simulink model "ctrl_TAPM"  (R2015a)
settings: Solver=ode3  StartTime=0.0  StopTime=inf  FixedStep=0.01  RelTol=1e-3
undefined symbols (not defined in the file): C, D, eps_c, epsilon, hd, hd2, I_s, k_cc, K_omega, K_q1f, K_q1r, K_q2f, K_q2r, K_q3f, K_q3r, K_q4f, K_q4r, K_q5f, K_q5r, K_q6f, K_q6r, K_T1f, K_T1r, K_T2f, K_T2r, K_T3f, K_T3r, K_T4f, K_T4r, K_T5f, K_T5r, K_T6f, K_T6r, Kp, Max_Acceleration, Max_rotation, Max_thrust, Min_thrust, n_c, n_max, p_cc, pwm_thr1_backward, pwm_thr1_forward, pwm_thr2_backward, pwm_thr2_forward, pwm_thr3_backward, pwm_thr3_forward, pwm_thr4_backward, pwm_thr4_forward, pwm_thr5_backward, pwm_thr5_forward, pwm_thr6_backward, pwm_thr6_forward, Q_f0, Q_max, r_cc, Rho, Thruster
libraries: marine_gnc x10, simulink x6, simulink_extras x3
(part 3 of 5)

== system ctrl_TAPM/Thruster control  ==
  "Desired thrust and angle " : Inport
  Delay : Delay  DelayLength=1  InitialCondition=0
  Demux : Demux  Outputs=12
  Mapping shaft speed and thrust : Selector  InputPortWidth=12  Indices="[1 7 2  8 3 9 4 10 5 11 6 12]"
  Mux : Mux  Inputs=12
  Mux1 : Mux  Inputs=2
  Selecting Desired thrust1 : Selector  InputPortWidth=12  Indices=[7 8 9 10 11 12]
  Selecting actual angle : Selector  InputPortWidth=12  Indices=[1 2 3 4 5 6]
  Subsystem1 : Subsystem
  Thrust and Shaft speed mapped to PWM : Subsystem
  Thruster 1 : Subsystem
      settings: AttributesFormatString=%<MinAlgLoopOccurrences>
  Thruster 2 : Subsystem
      settings: AttributesFormatString=%<MinAlgLoopOccurrences>
  Thruster 3 : Subsystem
      settings: AttributesFormatString=%<MinAlgLoopOccurrences>
  Thruster 4 : Subsystem
      settings: AttributesFormatString=%<MinAlgLoopOccurrences>
  Thruster 5 : Subsystem
      settings: AttributesFormatString=%<MinAlgLoopOccurrences>
  Thruster 6 : Subsystem
      settings: AttributesFormatString=%<MinAlgLoopOccurrences>
  "Commanded pwm " : Outport
  Commanded angle : Outport  Port=2
  Commanded thrust : Outport  Port=3
  wires:
  Selecting actual angle/1 -> Subsystem1/1(Calculated angles)
  "Desired thrust and angle "/1 -> Selecting actual angle/1, Selecting Desired thrust1/1
  Subsystem1/1(Commanded angles) -> Commanded angle/1
  Thrust and Shaft speed mapped to PWM/1(pwm) -> "Commanded pwm "/1
  Thrust and Shaft speed mapped to PWM/2(Force) -> Commanded thrust/1
  Thrust and Shaft speed mapped to PWM/3("Shaft speed ") -> Delay/1
  Thruster 1/1("Commanded thrust ") -> Mux/1
  Mux/1 -> Thrust and Shaft speed mapped to PWM/1(Calculated thrust)
  Mux1/1 -> Mapping shaft speed and thrust/1
  Delay/1 -> Mux1/2
  Mapping shaft speed and thrust/1 -> Demux/1
  Thruster 1/2(Shaft speed) -> Mux/2
  Demux/2 -> Thruster 1/2(shaft speed)
  Demux/1 -> Thruster 1/1(Desired thrust 1)
  Thruster 2/1("Commanded thrust ") -> Mux/3
  Demux/3 -> Thruster 2/1(Desired thrust 1)
  Demux/4 -> Thruster 2/2(shaft speed)
  Demux/5 -> Thruster 3/1(Desired thrust 1)
  Demux/6 -> Thruster 3/2(shaft speed)
  Demux/7 -> Thruster 4/1(Desired thrust 1)
  Demux/8 -> Thruster 4/2(shaft speed)
  Demux/9 -> Thruster 5/1(Desired thrust 1)
  Demux/10 -> Thruster 5/2(shaft speed)
  Demux/11 -> Thruster 6/1(Desired thrust 1)
  Demux/12 -> Thruster 6/2(shaft speed)
  Thruster 2/2(Shaft speed) -> Mux/4
  Thruster 3/1("Commanded thrust ") -> Mux/5
  Thruster 3/2(Shaft speed) -> Mux/6
  Thruster 4/1("Commanded thrust ") -> Mux/7
  Thruster 4/2(Shaft speed) -> Mux/8
  Thruster 5/1("Commanded thrust ") -> Mux/9
  Thruster 5/2(Shaft speed) -> Mux/10
  Thruster 6/1("Commanded thrust ") -> Mux/11
  Thruster 6/2(Shaft speed) -> Mux/12
  Selecting Desired thrust1/1 -> Mux1/1

== system ctrl_TAPM/Thruster measurment ==
  Mux1 : Mux  Inputs=6
  thr_angle_1 : S-Function  Priority=1  FunctionName=NIVeriStandIO  Parameters=width dtype portnum stime stype btype  mask(NI VeriStand Inport){portnum=1, width=-1, stime=-1, dtype=auto, stype=auto, btype=1}
      mask prompts: portnum "Port number:"; width "Port dimensions (-1 for dynamically sized):"; stime "Sample time (-1 for inherited):"; dtype "Data type:"; stype "Signal type:"; btype "Block type:"
      mask help: Use this inport on any level of nested subsystems to allow NI VeriStand software to map signals to it.
      mask init:
      | NIVeriStandIO_init;
      settings: CopyFcn=NIVeriStand_MDL_functions('', 'IO_copy');  DeleteFcn=NIVeriStand_MDL_functions('', 'IO_delete');  MoveFcn=set_param(gcb, 'Mask', 'on');
      mask Callback portnum: NIVeriStand_MDL_functions('', 'IO_setportnum');
      mask TypeOptions dtype: auto | double | single | int8 | uint8 | int16 | uint16 | int32 | uint32 | boolean
      mask Callback dtype: NIVeriStand_MDL_functions('', 'IO_booleansignal');
      mask TypeOptions stype: auto | real | complex
      mask Display:
      | patch([-x x], [-y y], [.90980 .81960 .32156]);
      | plot([xrad -x x xrad], [yrad -y y yrad]);
      | fprintf('NI In%d', portnum);
  thr_angle_2 : S-Function  Priority=2  FunctionName=NIVeriStandIO  Parameters=width dtype portnum stime stype btype  mask(NI VeriStand Inport){portnum=2, width=-1, stime=-1, dtype=auto, stype=auto, btype=1}
      mask prompts: portnum "Port number:"; width "Port dimensions (-1 for dynamically sized):"; stime "Sample time (-1 for inherited):"; dtype "Data type:"; stype "Signal type:"; btype "Block type:"
      mask help: Use this inport on any level of nested subsystems to allow NI VeriStand software to map signals to it.
      mask init:
      | NIVeriStandIO_init;
      settings: CopyFcn=NIVeriStand_MDL_functions('', 'IO_copy');  DeleteFcn=NIVeriStand_MDL_functions('', 'IO_delete');  MoveFcn=set_param(gcb, 'Mask', 'on');
      mask Callback portnum: NIVeriStand_MDL_functions('', 'IO_setportnum');
      mask TypeOptions dtype: auto | double | single | int8 | uint8 | int16 | uint16 | int32 | uint32 | boolean
      mask Callback dtype: NIVeriStand_MDL_functions('', 'IO_booleansignal');
      mask TypeOptions stype: auto | real | complex
      mask Display:
      | patch([-x x], [-y y], [.90980 .81960 .32156]);
      | plot([xrad -x x xrad], [yrad -y y yrad]);
      | fprintf('NI In%d', portnum);
  thr_angle_3 : S-Function  Priority=3  FunctionName=NIVeriStandIO  Parameters=width dtype portnum stime stype btype  mask(NI VeriStand Inport){portnum=3, width=-1, stime=-1, dtype=auto, stype=auto, btype=1}
      mask prompts: portnum "Port number:"; width "Port dimensions (-1 for dynamically sized):"; stime "Sample time (-1 for inherited):"; dtype "Data type:"; stype "Signal type:"; btype "Block type:"
      mask help: Use this inport on any level of nested subsystems to allow NI VeriStand software to map signals to it.
      mask init:
      | NIVeriStandIO_init;
      settings: CopyFcn=NIVeriStand_MDL_functions('', 'IO_copy');  DeleteFcn=NIVeriStand_MDL_functions('', 'IO_delete');  MoveFcn=set_param(gcb, 'Mask', 'on');
      mask Callback portnum: NIVeriStand_MDL_functions('', 'IO_setportnum');
      mask TypeOptions dtype: auto | double | single | int8 | uint8 | int16 | uint16 | int32 | uint32 | boolean
      mask Callback dtype: NIVeriStand_MDL_functions('', 'IO_booleansignal');
      mask TypeOptions stype: auto | real | complex
      mask Display:
      | patch([-x x], [-y y], [.90980 .81960 .32156]);
      | plot([xrad -x x xrad], [yrad -y y yrad]);
      | fprintf('NI In%d', portnum);
  thr_angle_4 : S-Function  Priority=4  FunctionName=NIVeriStandIO  Parameters=width dtype portnum stime stype btype  mask(NI VeriStand Inport){portnum=4, width=-1, stime=-1, dtype=auto, stype=auto, btype=1}
      mask prompts: portnum "Port number:"; width "Port dimensions (-1 for dynamically sized):"; stime "Sample time (-1 for inherited):"; dtype "Data type:"; stype "Signal type:"; btype "Block type:"
      mask help: Use this inport on any level of nested subsystems to allow NI VeriStand software to map signals to it.
      mask init:
      | NIVeriStandIO_init;
      settings: CopyFcn=NIVeriStand_MDL_functions('', 'IO_copy');  DeleteFcn=NIVeriStand_MDL_functions('', 'IO_delete');  MoveFcn=set_param(gcb, 'Mask', 'on');
      mask Callback portnum: NIVeriStand_MDL_functions('', 'IO_setportnum');
      mask TypeOptions dtype: auto | double | single | int8 | uint8 | int16 | uint16 | int32 | uint32 | boolean
      mask Callback dtype: NIVeriStand_MDL_functions('', 'IO_booleansignal');
      mask TypeOptions stype: auto | real | complex
      mask Display:
      | patch([-x x], [-y y], [.90980 .81960 .32156]);
      | plot([xrad -x x xrad], [yrad -y y yrad]);
      | fprintf('NI In%d', portnum);
  thr_angle_5 : S-Function  Priority=5  FunctionName=NIVeriStandIO  Parameters=width dtype portnum stime stype btype  mask(NI VeriStand Inport){portnum=5, width=-1, stime=-1, dtype=auto, stype=auto, btype=1}
      mask prompts: portnum "Port number:"; width "Port dimensions (-1 for dynamically sized):"; stime "Sample time (-1 for inherited):"; dtype "Data type:"; stype "Signal type:"; btype "Block type:"
      mask help: Use this inport on any level of nested subsystems to allow NI VeriStand software to map signals to it.
      mask init:
      | NIVeriStandIO_init;
      settings: CopyFcn=NIVeriStand_MDL_functions('', 'IO_copy');  DeleteFcn=NIVeriStand_MDL_functions('', 'IO_delete');  MoveFcn=set_param(gcb, 'Mask', 'on');
      mask Callback portnum: NIVeriStand_MDL_functions('', 'IO_setportnum');
      mask TypeOptions dtype: auto | double | single | int8 | uint8 | int16 | uint16 | int32 | uint32 | boolean
      mask Callback dtype: NIVeriStand_MDL_functions('', 'IO_booleansignal');
      mask TypeOptions stype: auto | real | complex
      mask Display:
      | patch([-x x], [-y y], [.90980 .81960 .32156]);
      | plot([xrad -x x xrad], [yrad -y y yrad]);
      | fprintf('NI In%d', portnum);
  thr_angle_6 : S-Function  Priority=6  FunctionName=NIVeriStandIO  Parameters=width dtype portnum stime stype btype  mask(NI VeriStand Inport){portnum=6, width=-1, stime=-1, dtype=auto, stype=auto, btype=1}
      mask prompts: portnum "Port number:"; width "Port dimensions (-1 for dynamically sized):"; stime "Sample time (-1 for inherited):"; dtype "Data type:"; stype "Signal type:"; btype "Block type:"
      mask help: Use this inport on any level of nested subsystems to allow NI VeriStand software to map signals to it.
      mask init:
      | NIVeriStandIO_init;
      settings: CopyFcn=NIVeriStand_MDL_functions('', 'IO_copy');  DeleteFcn=NIVeriStand_MDL_functions('', 'IO_delete');  MoveFcn=set_param(gcb, 'Mask', 'on');
      mask Callback portnum: NIVeriStand_MDL_functions('', 'IO_setportnum');
      mask TypeOptions dtype: auto | double | single | int8 | uint8 | int16 | uint16 | int32 | uint32 | boolean
      mask Callback dtype: NIVeriStand_MDL_functions('', 'IO_booleansignal');
      mask TypeOptions stype: auto | real | complex
      mask Display:
      | patch([-x x], [-y y], [.90980 .81960 .32156]);
      | plot([xrad -x x xrad], [yrad -y y yrad]);
      | fprintf('NI In%d', portnum);
  alpha_m : Outport
  wires:
  thr_angle_3/1 -> Mux1/3
  thr_angle_1/1 -> Mux1/1
  Mux1/1 -> alpha_m/1
  thr_angle_5/1 -> Mux1/5
  thr_angle_4/1 -> Mux1/4
  thr_angle_6/1 -> Mux1/6
  thr_angle_2/1 -> Mux1/2

== system ctrl_TAPM/IMU/Wild point cleaner ==
  Y : Inport
  MATLAB Function : MATLAB Function  TreatAsAtomicUnit=on
  Memory : Memory  X0=[4.968, 4.965, 4.97, 4.975, 4.96]
  Memory1 : Memory  X0=[0, 0, 0, 0, 0, 0, 0]
  Y_filtered : Outport
  wires:
  Y/1 -> MATLAB Function/2(Y)
  MATLAB Function/2(Y_filtered) -> Memory1/1, Y_filtered/1
  MATLAB Function/1(V_hist1) -> Memory/1
  Memory/1 -> MATLAB Function/1(V_hist)
  Memory1/1 -> MATLAB Function/3(Y_prev)

== system ctrl_TAPM/IMU/Wild point cleaner1 ==
  Y : Inport
  MATLAB Function : MATLAB Function  TreatAsAtomicUnit=on
  Memory : Memory  X0=[4.968, 4.965, 4.97, 4.975, 4.96]
  Memory1 : Memory  X0=[0, 0, 0, 0, 0, 0, 0]
  Y_filtered : Outport
  wires:
  Y/1 -> MATLAB Function/2(Y)
  MATLAB Function/2(Y_filtered) -> Memory1/1, Y_filtered/1
  MATLAB Function/1(V_hist1) -> Memory/1
  Memory/1 -> MATLAB Function/1(V_hist)
  Memory1/1 -> MATLAB Function/3(Y_prev)

== system ctrl_TAPM/TAPM Controller w_observer/LQR ==
  SP : Inport
  eta : Inport  Port=2
  bias : Inport  Port=3
  Constant : Constant
  Delay : Delay  DelayLength=1  InitialCondition=0
  Integrator : Integrator  ExternalReset=rising  IgnoreLimit=on
  MATLAB Function : MATLAB Function  TreatAsAtomicUnit=on
  MATLAB Function1 : MATLAB Function  TreatAsAtomicUnit=on
  MATLAB Function2 : MATLAB Function  TreatAsAtomicUnit=on
  MATLAB Function3 : MATLAB Function  TreatAsAtomicUnit=on
  Multiport Switch : MultiPortSwitch  Inputs=2
  controller : S-Function  Priority=1  FunctionName=NIVeriStandIO  Parameters=width dtype portnum stime stype btype  mask(NI VeriStand Outport){portnum=1, width=-1, stime=-1, dtype=auto, stype=auto, btype=0}
      mask prompts: portnum "Port number:"; width "Port dimensions (-1 for dynamically sized):"; stime "Sample time (-1 for inherited):"; dtype "Data type:"; stype "Signal type:"; btype "Block type:"
      mask help: Use this outport on any level of nested subsystems to allow NI VeriStand software to map signals to it.
      mask init:
      | NIVeriStandIO_init;
      settings: CopyFcn=NIVeriStand_MDL_functions('', 'IO_copy');  DeleteFcn=NIVeriStand_MDL_functions('', 'IO_delete');  MoveFcn=set_param(gcb, 'Mask', 'on');
      mask Callback portnum: NIVeriStand_MDL_functions('', 'IO_setportnum');
      mask TypeOptions dtype: auto | double | single | int8 | uint8 | int16 | uint16 | int32 | uint32 | boolean
      mask Callback dtype: NIVeriStand_MDL_functions('', 'IO_booleansignal');
      mask TypeOptions stype: auto | real | complex
      mask Display:
      | patch([-x x], [-y y], [.90980 .81960 .32156]);
      | plot([xrad -x x xrad], [yrad -y y yrad]);
      | fprintf('NI Out%d', portnum);
  timer : S-Function  Priority=2  FunctionName=NIVeriStandIO  Parameters=width dtype portnum stime stype btype  mask(NI VeriStand Outport){portnum=2, width=-1, stime=-1, dtype=auto, stype=auto, btype=0}
      mask prompts: portnum "Port number:"; width "Port dimensions (-1 for dynamically sized):"; stime "Sample time (-1 for inherited):"; dtype "Data type:"; stype "Signal type:"; btype "Block type:"
      mask help: Use this outport on any level of nested subsystems to allow NI VeriStand software to map signals to it.
      mask init:
      | NIVeriStandIO_init;
      settings: CopyFcn=NIVeriStand_MDL_functions('', 'IO_copy');  DeleteFcn=NIVeriStand_MDL_functions('', 'IO_delete');  MoveFcn=set_param(gcb, 'Mask', 'on');
      mask Callback portnum: NIVeriStand_MDL_functions('', 'IO_setportnum');
      mask TypeOptions dtype: auto | double | single | int8 | uint8 | int16 | uint16 | int32 | uint32 | boolean
      mask Callback dtype: NIVeriStand_MDL_functions('', 'IO_booleansignal');
      mask TypeOptions stype: auto | real | complex
      mask Display:
      | patch([-x x], [-y y], [.90980 .81960 .32156]);
      | plot([xrad -x x xrad], [yrad -y y yrad]);
      | fprintf('NI Out%d', portnum);
  tau_d : Outport  PortDimensions=3
  wires:
  SP/1 -> MATLAB Function3/1(r), MATLAB Function1/1(r)
  eta/1 -> MATLAB Function/3(eta), MATLAB Function1/2(x_hat), MATLAB Function3/2(x_hat)
  Constant/1 -> Integrator/1
  MATLAB Function/1(reset) -> Integrator/2
  Integrator/1 -> Delay/1
  MATLAB Function/2(y) -> controller/1, Multiport Switch/1
  Delay/1 -> timer/1, MATLAB Function/1(timer)
  bias/1 -> MATLAB Function1/3(bias), MATLAB Function3/3(bias)
  [r_max] -> MATLAB Function/2(rmax)
  Multiport Switch/1 -> MATLAB Function2/1(u)
  MATLAB Function1/1(tau) -> Multiport Switch/2
  MATLAB Function3/1(tau) -> Multiport Switch/3
  MATLAB Function2/1(y) -> tau_d/1

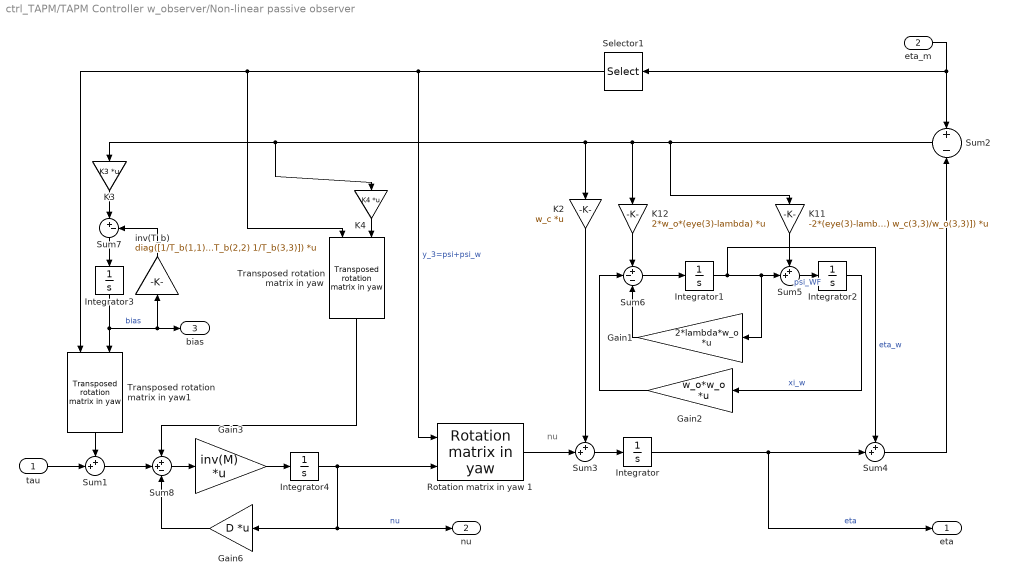
== system ctrl_TAPM/TAPM Controller w_observer/Non-linear passive observer  ==
  note: nu
  tau : Inport
  eta_m : Inport  Port=2
  Gain1 : Gain  Gain=2*lambda*w_o  Multiplication=Matrix(K*u)  SaturateOnIntegerOverflow=on  OutDataTypeStr=Inherit: Same as input  ParamDataTypeStr=Inherit: Same as input
  Gain2 : Gain  Gain=w_o*w_o  Multiplication=Matrix(K*u)  SaturateOnIntegerOverflow=on  OutDataTypeStr=Inherit: Same as input  ParamDataTypeStr=Inherit: Same as input
  Gain3 : Gain  Gain=inv(M)  Multiplication=Matrix(K*u)  SaturateOnIntegerOverflow=on  OutDataTypeStr=Inherit: Same as input  ParamDataTypeStr=Inherit: Same as input
  Gain6 : Gain  Gain=D  Multiplication=Matrix(K*u)  SaturateOnIntegerOverflow=on  OutDataTypeStr=Inherit: Same as input  ParamDataTypeStr=Inherit: Same as input
  Integrator : Integrator  InitialCondition=[0,0,0]'
  Integrator1 : Integrator
  Integrator2 : Integrator
  Integrator3 : Integrator
  Integrator4 : Integrator  InitialCondition=[0,0,0]'
  K11 : Gain  Gain=-2*(eye(3)-lambda)*diag([w_c(1,1)/w_o(1,1) w_c(2,2)/w_o(2,2) w_c(3,3)/w_o(3,3)])  Multiplication=Matrix(K*u)  SaturateOnIntegerOverflow=on  OutDataTypeStr=Inherit: Same as input  ParamDataTypeStr=Inherit: Same as input
  K12 : Gain  Gain=2*w_o*(eye(3)-lambda)  Multiplication=Matrix(K*u)  SaturateOnIntegerOverflow=on  OutDataTypeStr=Inherit: Same as input  ParamDataTypeStr=Inherit: Same as input
  K2 : Gain  Gain=w_c  Multiplication=Matrix(K*u)  SaturateOnIntegerOverflow=on  OutDataTypeStr=Inherit: Same as input  ParamDataTypeStr=Inherit: Same as input
  K3 : Gain  Gain=K3  Multiplication=Matrix(K*u)  SaturateOnIntegerOverflow=on  OutDataTypeStr=Inherit: Same as input  ParamDataTypeStr=Inherit: Same as input
  K4 : Gain  Gain=K4  Multiplication=Matrix(K*u)  SaturateOnIntegerOverflow=on  OutDataTypeStr=Inherit: Same as input  ParamDataTypeStr=Inherit: Same as input
  Rotation matrix in yaw 1 : marine_gnc/Models/ Kinematics/Rotation matrix in yaw 
  Selector1 : Selector  InputPortWidth=3  Indices=[3]
  Sum{1,3..5} (4 alike) : Sum  Inputs=++|  SaturateOnIntegerOverflow=on  InputSameDT=on  OutDataTypeStr=Inherit: Same as first input
  Sum2 : Sum  Inputs=+|-  SaturateOnIntegerOverflow=on  InputSameDT=on  OutDataTypeStr=Inherit: Same as first input
  Sum6 : Sum  Inputs=+--  SaturateOnIntegerOverflow=on  InputSameDT=on  OutDataTypeStr=Inherit: Same as first input
  Sum7 : Sum  Inputs=|+-  SaturateOnIntegerOverflow=on  InputSameDT=on  OutDataTypeStr=Inherit: Same as first input
  Sum8 : Sum  Inputs=++-  SaturateOnIntegerOverflow=on  InputSameDT=on  OutDataTypeStr=Inherit: Same as first input
  Transposed rotation matrix in yaw : marine_gnc/Models/ Kinematics/Transposed rotation  matrix in yaw
  Transposed rotation matrix in yaw1 : marine_gnc/Models/ Kinematics/Transposed rotation  matrix in yaw
  inv(T_b) : Gain  Gain=diag([1/T_b(1,1) 1/T_b(2,2) 1/T_b(3,3)])  Multiplication=Matrix(K*u)  SaturateOnIntegerOverflow=on  OutDataTypeStr=Inherit: Same as input  ParamDataTypeStr=Inherit: Same as input
  eta : Outport
  nu : Outport  Port=2
  bias : Outport  Port=3  PortDimensions=3
  wires:
  Sum3/1 -> Integrator/1
  Integrator2/1 -> Gain2/1  "xi_w"
  Gain2/1 -> Sum6/2
  Sum6/1 -> Integrator1/1
  Sum4/1 -> Sum2/2
  Sum2/1 -> K4/1, K3/1, K2/1, K12/1, K11/1
  Gain1/1 -> Sum6/3
  K2/1 -> Sum3/1
  Integrator/1 -> Sum4/2, eta/1  "eta"
  inv(T_b)/1 -> Sum7/2
  Integrator3/1 -> Transposed rotation matrix in yaw1/2, bias/1, inv(T_b)/1  "bias"
  tau/1 -> Sum1/2
  Integrator1/1 -> Sum4/1, Gain1/1, Sum5/2  "eta_w"
  K12/1 -> Sum6/1
  K11/1 -> Sum5/1
  eta_m/1 -> Selector1/1, Sum2/1
  Sum5/1 -> Integrator2/1  "psi_WF"
  Sum7/1 -> Integrator3/1
  Sum1/1 -> Sum8/2
  Rotation matrix in yaw 1/1 -> Sum3/2
  K3/1 -> Sum7/1
  Selector1/1 -> Transposed rotation matrix in yaw1/1, Transposed rotation matrix in yaw/1, Rotation matrix in yaw 1/1  "y_3=psi+psi_w"
  Gain3/1 -> Integrator4/1
  Sum8/1 -> Gain3/1
  Integrator4/1 -> nu/1, Gain6/1, Rotation matrix in yaw 1/2  "nu"
  Transposed rotation matrix in yaw1/1 -> Sum1/1
  Transposed rotation matrix in yaw/1 -> Sum8/1
  K4/1 -> Transposed rotation matrix in yaw/2
  Gain6/1 -> Sum8/3

== system ctrl_TAPM/TAPM Controller w_observer/PID ==
  eta_ref : Inport
  eta : Inport  Port=2
  nu : Inport  Port=3
  Constant : Constant
  DP controller : Subsystem  AncestorBlock="marine_gnc/Control/Dynamic  Positioning /DP controller"
  DP controller1 : Subsystem  AncestorBlock="marine_gnc/Control/Dynamic  Positioning /DP controller"
  Delay : Delay  DelayLength=1  InitialCondition=0
  Integrator : Integrator  ExternalReset=rising  IgnoreLimit=on
  MATLAB Function : MATLAB Function  TreatAsAtomicUnit=on
  Multiport Switch : MultiPortSwitch  Inputs=2
  controller : S-Function  Priority=1  FunctionName=NIVeriStandIO  Parameters=width dtype portnum stime stype btype  mask(NI VeriStand Outport){portnum=1, width=-1, stime=-1, dtype=auto, stype=auto, btype=0}
      mask prompts: portnum "Port number:"; width "Port dimensions (-1 for dynamically sized):"; stime "Sample time (-1 for inherited):"; dtype "Data type:"; stype "Signal type:"; btype "Block type:"
      mask help: Use this outport on any level of nested subsystems to allow NI VeriStand software to map signals to it.
      mask init:
      | NIVeriStandIO_init;
      settings: CopyFcn=NIVeriStand_MDL_functions('', 'IO_copy');  DeleteFcn=NIVeriStand_MDL_functions('', 'IO_delete');  MoveFcn=set_param(gcb, 'Mask', 'on');
      mask Callback portnum: NIVeriStand_MDL_functions('', 'IO_setportnum');
      mask TypeOptions dtype: auto | double | single | int8 | uint8 | int16 | uint16 | int32 | uint32 | boolean
      mask Callback dtype: NIVeriStand_MDL_functions('', 'IO_booleansignal');
      mask TypeOptions stype: auto | real | complex
      mask Display:
      | patch([-x x], [-y y], [.90980 .81960 .32156]);
      | plot([xrad -x x xrad], [yrad -y y yrad]);
      | fprintf('NI Out%d', portnum);
  timer : S-Function  Priority=2  FunctionName=NIVeriStandIO  Parameters=width dtype portnum stime stype btype  mask(NI VeriStand Outport){portnum=2, width=-1, stime=-1, dtype=auto, stype=auto, btype=0}
      mask prompts: portnum "Port number:"; width "Port dimensions (-1 for dynamically sized):"; stime "Sample time (-1 for inherited):"; dtype "Data type:"; stype "Signal type:"; btype "Block type:"
      mask help: Use this outport on any level of nested subsystems to allow NI VeriStand software to map signals to it.
      mask init:
      | NIVeriStandIO_init;
      settings: CopyFcn=NIVeriStand_MDL_functions('', 'IO_copy');  DeleteFcn=NIVeriStand_MDL_functions('', 'IO_delete');  MoveFcn=set_param(gcb, 'Mask', 'on');
      mask Callback portnum: NIVeriStand_MDL_functions('', 'IO_setportnum');
      mask TypeOptions dtype: auto | double | single | int8 | uint8 | int16 | uint16 | int32 | uint32 | boolean
      mask Callback dtype: NIVeriStand_MDL_functions('', 'IO_booleansignal');
      mask TypeOptions stype: auto | real | complex
      mask Display:
      | patch([-x x], [-y y], [.90980 .81960 .32156]);
      | plot([xrad -x x xrad], [yrad -y y yrad]);
      | fprintf('NI Out%d', portnum);
  tau : Outport
  wires:
  DP controller/1(tau) -> Multiport Switch/2
  nu/1 -> DP controller1/3(nu), DP controller/3(nu)
  eta_ref/1 -> DP controller1/1(eta_ref), DP controller/1(eta_ref)
  eta/1 -> DP controller1/2(eta), MATLAB Function/3(eta), DP controller/2(eta)
  Constant/1 -> Integrator/1
  MATLAB Function/1(reset) -> Integrator/2
  Integrator/1 -> Delay/1
  MATLAB Function/2(y) -> controller/1, Multiport Switch/1
  Delay/1 -> timer/1, MATLAB Function/1(timer)
  [r_max] -> MATLAB Function/2(rmax)
  Multiport Switch/1 -> tau/1
  DP controller1/1(tau) -> Multiport Switch/3

== system ctrl_TAPM/TAPM Controller w_observer/SP Generator ==
  eta : Inport
  wave_dir : Inport  Port=2
  Constant1 : Constant  Value=pi
  Gain : Gain  Gain=diag([1/(1/sqrt(90)) 1/(1/sqrt(90))])  Multiplication=Matrix(K*u)
  Gain1 : Gain  Gain=diag([1/(1/sqrt(90)) 1/(1/sqrt(90))])  Multiplication=Matrix(K*u)
  Integrator : Integrator  InitialCondition=[0 0]
  Mux : Mux  Inputs=2
  Selector : Selector  InputPortWidth=3  Indices=[1 2]
  Set-Point Limiter : MATLAB Function  TreatAsAtomicUnit=on
  Sum : Sum  Inputs=|++
  Sum1 : Sum  Inputs=|+-
  Transfer Fcn2 : TransferFcn  Denominator=[0.5 1]
  SP : Outport  PortDimensions=3
  wires:
  Integrator/1 -> Gain/1, Set-Point Limiter/1(sp)
  [fzp] -> Set-Point Limiter/2(fzp)
  [r_max] -> Set-Point Limiter/3(rmax)
  Mux/1 -> SP/1
  eta/1 -> Selector/1
  Transfer Fcn2/1 -> Mux/2
  Constant1/1 -> Sum/1
  Sum/1 -> Transfer Fcn2/1
  wave_dir/1 -> Sum/2
  Set-Point Limiter/1(sp_new) -> Mux/1
  Sum1/1 -> Integrator/1
  Selector/1 -> Gain1/1
  Gain/1 -> Sum1/2
  Gain1/1 -> Sum1/1

== system ctrl_TAPM/Thrust allocation/Optimal angle path and constraints on rotation speed ==
  Desired Angle : Inport  Partition=on  PartitionDimension=1  PartitionWidth=1
  "initial angle " : Inport  Port=2  Partition=on  PartitionDimension=1  PartitionWidth=1
  reset : Inport  Port=3  Partition=on  PartitionDimension=1  PartitionWidth=1
  Degrees to Radians : simulink_extras/Transformations/Degrees to Radians
  Delay : Delay  DelayLength=1  InitialCondition=0
  Discrete-Time Integrator : DiscreteIntegrator  ExternalReset=either  InitialConditionSource=external  InitialConditionSetting=State (most efficient)  SampleTime=0.01
  Ensuring angle is [-pi pi] : MATLAB Function  TreatAsAtomicUnit=on
  For Each : ForEach  DisableCoverage=on  IndexMode=One-based
  MATLAB Function1 : MATLAB Function  TreatAsAtomicUnit=on
  Max Rotation Rate : Saturate  UpperLimit=Max_rotation  LowerLimit=-Max_rotation
  commanded Angle : Outport  ConcatenationDimension=1
  wires:
  Degrees to Radians/1 -> Ensuring angle is [-pi pi]/1(angle)
  Ensuring angle is [-pi pi]/1(y) -> commanded Angle/1
  Discrete-Time Integrator/1 -> Degrees to Radians/1, Delay/1  "angle"
  "initial angle "/1 -> Discrete-Time Integrator/3
  Max Rotation Rate/1 -> Discrete-Time Integrator/1
  MATLAB Function1/1(psi_D) -> Max Rotation Rate/1
  Desired Angle/1 -> MATLAB Function1/1(desired)
  reset/1 -> Discrete-Time Integrator/2
  Delay/1 -> MATLAB Function1/2(actual)

== system ctrl_TAPM/Thruster control /Subsystem1 ==
  Calculated angles : Inport
  Demux : Demux  Outputs=6
  Mux : Mux  Inputs=6
  Saturation {1..6} (6 alike) : Saturate  UpperLimit=pi  LowerLimit=-pi
  Commanded angles : Outport
  wires:
  Calculated angles/1 -> Demux/1
  Demux/1 -> Saturation 1/1
  Demux/2 -> Saturation 2/1
  Demux/3 -> Saturation 3/1
  Demux/4 -> Saturation 4/1
  Demux/5 -> Saturation 5/1
  Demux/6 -> Saturation 6/1
  Mux/1 -> Commanded angles/1
  Saturation 1/1 -> Mux/1
  Saturation 6/1 -> Mux/6
  Saturation 5/1 -> Mux/5
  Saturation 2/1 -> Mux/2
  Saturation 3/1 -> Mux/3
  Saturation 4/1 -> Mux/4

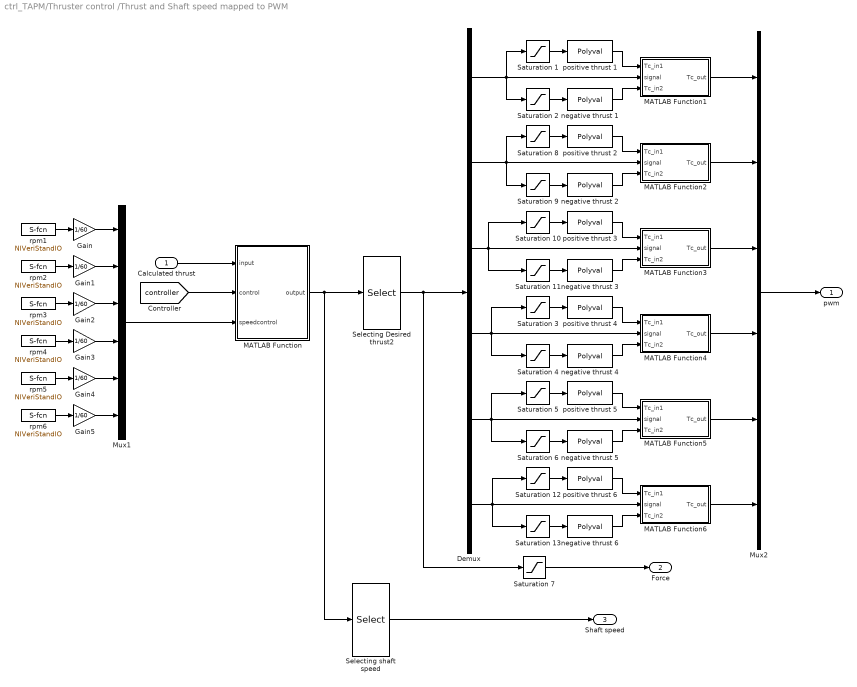
== system ctrl_TAPM/Thruster control /Thrust and Shaft speed mapped to PWM ==
  Calculated thrust : Inport
  Demux : Demux  Outputs=6
  Gain{,1..5} (6 alike) : Gain  Gain=1/60
  MATLAB Function : MATLAB Function  TreatAsAtomicUnit=on
  MATLAB Function1 : MATLAB Function  TreatAsAtomicUnit=on
  MATLAB Function2 : MATLAB Function  TreatAsAtomicUnit=on
  MATLAB Function3 : MATLAB Function  TreatAsAtomicUnit=on
  MATLAB Function4 : MATLAB Function  TreatAsAtomicUnit=on
  MATLAB Function5 : MATLAB Function  TreatAsAtomicUnit=on
  MATLAB Function6 : MATLAB Function  TreatAsAtomicUnit=on
  Mux1 : Mux  Inputs=6
  Mux2 : Mux  Inputs=6
  Saturation {1,3,5,8,10,12} (6 alike) : Saturate  UpperLimit=Max_thrust  LowerLimit=0
  Saturation {2,4,6,9,11,13} (6 alike) : Saturate  UpperLimit=0  LowerLimit=Min_thrust
  Saturation 7 : Saturate  UpperLimit=Max_thrust  LowerLimit=-Max_thrust
  Selecting Desired thrust2 : Selector  InputPortWidth=12  Indices=[1 3 5 7 9 11]
  Selecting shaft speed : Selector  InputPortWidth=12  Indices=[2 4 6 8 10 12]
  negative thrust 1 : Polyval  Coefs=pwm_thr1_backward
  negative thrust 2 : Polyval  Coefs=pwm_thr2_backward
  negative thrust 3 : Polyval  Coefs=pwm_thr3_backward
  negative thrust 4 : Polyval  Coefs=pwm_thr4_backward
  negative thrust 5 : Polyval  Coefs=pwm_thr5_backward
  negative thrust 6 : Polyval  Coefs=pwm_thr6_backward
  positive thrust 1 : Polyval  Coefs=pwm_thr1_forward
  positive thrust 2 : Polyval  Coefs=pwm_thr2_forward
  positive thrust 3 : Polyval  Coefs=pwm_thr3_forward
  positive thrust 4 : Polyval  Coefs=pwm_thr4_forward
  positive thrust 5 : Polyval  Coefs=pwm_thr5_forward
  positive thrust 6 : Polyval  Coefs=pwm_thr6_forward
  "rpm1 " : S-Function  Priority=1  FunctionName=NIVeriStandIO  Parameters=width dtype portnum stime stype btype  mask(NI VeriStand Inport){portnum=1, width=-1, stime=-1, dtype=auto, stype=auto, btype=1}
      mask prompts: portnum "Port number:"; width "Port dimensions (-1 for dynamically sized):"; stime "Sample time (-1 for inherited):"; dtype "Data type:"; stype "Signal type:"; btype "Block type:"
      mask help: Use this inport on any level of nested subsystems to allow NI VeriStand software to map signals to it.
      mask init:
      | NIVeriStandIO_init;
      settings: CopyFcn=NIVeriStand_MDL_functions('', 'IO_copy');  DeleteFcn=NIVeriStand_MDL_functions('', 'IO_delete');  MoveFcn=set_param(gcb, 'Mask', 'on');
      mask Callback portnum: NIVeriStand_MDL_functions('', 'IO_setportnum');
      mask TypeOptions dtype: auto | double | single | int8 | uint8 | int16 | uint16 | int32 | uint32 | boolean
      mask Callback dtype: NIVeriStand_MDL_functions('', 'IO_booleansignal');
      mask TypeOptions stype: auto | real | complex
      mask Display:
      | patch([-x x], [-y y], [.90980 .81960 .32156]);
      | plot([xrad -x x xrad], [yrad -y y yrad]);
      | fprintf('NI In%d', portnum);
  rpm2 : S-Function  Priority=2  FunctionName=NIVeriStandIO  Parameters=width dtype portnum stime stype btype  mask(NI VeriStand Inport){portnum=2, width=-1, stime=-1, dtype=auto, stype=auto, btype=1}
      mask prompts: portnum "Port number:"; width "Port dimensions (-1 for dynamically sized):"; stime "Sample time (-1 for inherited):"; dtype "Data type:"; stype "Signal type:"; btype "Block type:"
      mask help: Use this inport on any level of nested subsystems to allow NI VeriStand software to map signals to it.
      mask init:
      | NIVeriStandIO_init;
      settings: CopyFcn=NIVeriStand_MDL_functions('', 'IO_copy');  DeleteFcn=NIVeriStand_MDL_functions('', 'IO_delete');  MoveFcn=set_param(gcb, 'Mask', 'on');
      mask Callback portnum: NIVeriStand_MDL_functions('', 'IO_setportnum');
      mask TypeOptions dtype: auto | double | single | int8 | uint8 | int16 | uint16 | int32 | uint32 | boolean
      mask Callback dtype: NIVeriStand_MDL_functions('', 'IO_booleansignal');
      mask TypeOptions stype: auto | real | complex
      mask Display:
      | patch([-x x], [-y y], [.90980 .81960 .32156]);
      | plot([xrad -x x xrad], [yrad -y y yrad]);
      | fprintf('NI In%d', portnum);
  rpm3 : S-Function  Priority=3  FunctionName=NIVeriStandIO  Parameters=width dtype portnum stime stype btype  mask(NI VeriStand Inport){portnum=3, width=-1, stime=-1, dtype=auto, stype=auto, btype=1}
      mask prompts: portnum "Port number:"; width "Port dimensions (-1 for dynamically sized):"; stime "Sample time (-1 for inherited):"; dtype "Data type:"; stype "Signal type:"; btype "Block type:"
      mask help: Use this inport on any level of nested subsystems to allow NI VeriStand software to map signals to it.
      mask init:
      | NIVeriStandIO_init;
      settings: CopyFcn=NIVeriStand_MDL_functions('', 'IO_copy');  DeleteFcn=NIVeriStand_MDL_functions('', 'IO_delete');  MoveFcn=set_param(gcb, 'Mask', 'on');
      mask Callback portnum: NIVeriStand_MDL_functions('', 'IO_setportnum');
      mask TypeOptions dtype: auto | double | single | int8 | uint8 | int16 | uint16 | int32 | uint32 | boolean
      mask Callback dtype: NIVeriStand_MDL_functions('', 'IO_booleansignal');
      mask TypeOptions stype: auto | real | complex
      mask Display:
      | patch([-x x], [-y y], [.90980 .81960 .32156]);
      | plot([xrad -x x xrad], [yrad -y y yrad]);
      | fprintf('NI In%d', portnum);
  rpm4 : S-Function  Priority=4  FunctionName=NIVeriStandIO  Parameters=width dtype portnum stime stype btype  mask(NI VeriStand Inport){portnum=4, width=-1, stime=-1, dtype=auto, stype=auto, btype=1}
      mask prompts: portnum "Port number:"; width "Port dimensions (-1 for dynamically sized):"; stime "Sample time (-1 for inherited):"; dtype "Data type:"; stype "Signal type:"; btype "Block type:"
      mask help: Use this inport on any level of nested subsystems to allow NI VeriStand software to map signals to it.
      mask init:
      | NIVeriStandIO_init;
      settings: CopyFcn=NIVeriStand_MDL_functions('', 'IO_copy');  DeleteFcn=NIVeriStand_MDL_functions('', 'IO_delete');  MoveFcn=set_param(gcb, 'Mask', 'on');
      mask Callback portnum: NIVeriStand_MDL_functions('', 'IO_setportnum');
      mask TypeOptions dtype: auto | double | single | int8 | uint8 | int16 | uint16 | int32 | uint32 | boolean
      mask Callback dtype: NIVeriStand_MDL_functions('', 'IO_booleansignal');
      mask TypeOptions stype: auto | real | complex
      mask Display:
      | patch([-x x], [-y y], [.90980 .81960 .32156]);
      | plot([xrad -x x xrad], [yrad -y y yrad]);
      | fprintf('NI In%d', portnum);
  rpm5 : S-Function  Priority=5  FunctionName=NIVeriStandIO  Parameters=width dtype portnum stime stype btype  mask(NI VeriStand Inport){portnum=5, width=-1, stime=-1, dtype=auto, stype=auto, btype=1}
      mask prompts: portnum "Port number:"; width "Port dimensions (-1 for dynamically sized):"; stime "Sample time (-1 for inherited):"; dtype "Data type:"; stype "Signal type:"; btype "Block type:"
      mask help: Use this inport on any level of nested subsystems to allow NI VeriStand software to map signals to it.
      mask init:
      | NIVeriStandIO_init;
      settings: CopyFcn=NIVeriStand_MDL_functions('', 'IO_copy');  DeleteFcn=NIVeriStand_MDL_functions('', 'IO_delete');  MoveFcn=set_param(gcb, 'Mask', 'on');
      mask Callback portnum: NIVeriStand_MDL_functions('', 'IO_setportnum');
      mask TypeOptions dtype: auto | double | single | int8 | uint8 | int16 | uint16 | int32 | uint32 | boolean
      mask Callback dtype: NIVeriStand_MDL_functions('', 'IO_booleansignal');
      mask TypeOptions stype: auto | real | complex
      mask Display:
      | patch([-x x], [-y y], [.90980 .81960 .32156]);
      | plot([xrad -x x xrad], [yrad -y y yrad]);
      | fprintf('NI In%d', portnum);
  rpm6 : S-Function  Priority=6  FunctionName=NIVeriStandIO  Parameters=width dtype portnum stime stype btype  mask(NI VeriStand Inport){portnum=6, width=-1, stime=-1, dtype=auto, stype=auto, btype=1}
      mask prompts: portnum "Port number:"; width "Port dimensions (-1 for dynamically sized):"; stime "Sample time (-1 for inherited):"; dtype "Data type:"; stype "Signal type:"; btype "Block type:"
      mask help: Use this inport on any level of nested subsystems to allow NI VeriStand software to map signals to it.
      mask init:
      | NIVeriStandIO_init;
      settings: CopyFcn=NIVeriStand_MDL_functions('', 'IO_copy');  DeleteFcn=NIVeriStand_MDL_functions('', 'IO_delete');  MoveFcn=set_param(gcb, 'Mask', 'on');
      mask Callback portnum: NIVeriStand_MDL_functions('', 'IO_setportnum');
      mask TypeOptions dtype: auto | double | single | int8 | uint8 | int16 | uint16 | int32 | uint32 | boolean
      mask Callback dtype: NIVeriStand_MDL_functions('', 'IO_booleansignal');
      mask TypeOptions stype: auto | real | complex
      mask Display:
      | patch([-x x], [-y y], [.90980 .81960 .32156]);
      | plot([xrad -x x xrad], [yrad -y y yrad]);
      | fprintf('NI In%d', portnum);
  pwm : Outport
  Force : Outport  Port=2
  "Shaft speed " : Outport  Port=3
  wires:
  MATLAB Function/1(output) -> Selecting shaft speed/1, Selecting Desired thrust2/1
  [controller] -> MATLAB Function/2(control)
  Mux2/1 -> pwm/1
  Selecting Desired thrust2/1 -> Saturation 7/1, Demux/1
  Selecting shaft speed/1 -> "Shaft speed "/1
  Saturation 7/1 -> Force/1
  "rpm1 "/1 -> Gain/1
  rpm2/1 -> Gain1/1
  rpm3/1 -> Gain2/1
  rpm4/1 -> Gain3/1
  rpm5/1 -> Gain4/1
  rpm6/1 -> Gain5/1
  Mux1/1 -> MATLAB Function/3(speedcontrol)
  positive thrust 1/1 -> MATLAB Function1/1(Tc_in1)
  negative thrust 1/1 -> MATLAB Function1/3(Tc_in2)
  Demux/1 -> Saturation 1/1, MATLAB Function1/2(signal), Saturation 2/1
  MATLAB Function1/1(Tc_out) -> Mux2/1
  Saturation 1/1 -> positive thrust 1/1
  Saturation 2/1 -> negative thrust 1/1
  positive thrust 2/1 -> MATLAB Function2/1(Tc_in1)
  negative thrust 2/1 -> MATLAB Function2/3(Tc_in2)
  Demux/2 -> Saturation 9/1, Saturation 8/1, MATLAB Function2/2(signal)
  MATLAB Function2/1(Tc_out) -> Mux2/2
  Saturation 8/1 -> positive thrust 2/1
  Saturation 9/1 -> negative thrust 2/1
  positive thrust 3/1 -> MATLAB Function3/1(Tc_in1)
  negative thrust 3/1 -> MATLAB Function3/3(Tc_in2)
  Demux/3 -> Saturation 11/1, MATLAB Function3/2(signal), Saturation 10/1
  MATLAB Function3/1(Tc_out) -> Mux2/3
  Saturation 10/1 -> positive thrust 3/1
  Saturation 11/1 -> negative thrust 3/1
  positive thrust 4/1 -> MATLAB Function4/1(Tc_in1)
  negative thrust 4/1 -> MATLAB Function4/3(Tc_in2)
  MATLAB Function4/1(Tc_out) -> Mux2/4
  Saturation 3/1 -> positive thrust 4/1
  Saturation 4/1 -> negative thrust 4/1
  Demux/4 -> Saturation 3/1, Saturation 4/1, MATLAB Function4/2(signal)
  positive thrust 5/1 -> MATLAB Function5/1(Tc_in1)
  negative thrust 5/1 -> MATLAB Function5/3(Tc_in2)
  MATLAB Function5/1(Tc_out) -> Mux2/5
  Saturation 5/1 -> positive thrust 5/1
  Saturation 6/1 -> negative thrust 5/1
  Demux/5 -> Saturation 5/1, MATLAB Function5/2(signal), Saturation 6/1
  positive thrust 6/1 -> MATLAB Function6/1(Tc_in1)
  negative thrust 6/1 -> MATLAB Function6/3(Tc_in2)
  MATLAB Function6/1(Tc_out) -> Mux2/6
  Saturation 12/1 -> positive thrust 6/1
  Saturation 13/1 -> negative thrust 6/1
  Demux/6 -> Saturation 13/1, Saturation 12/1, MATLAB Function6/2(signal)
  Gain/1 -> Mux1/1
  Gain5/1 -> Mux1/6
  Gain4/1 -> Mux1/5
  Gain3/1 -> Mux1/4
  Gain2/1 -> Mux1/3
  Gain1/1 -> Mux1/2
  Calculated thrust/1 -> MATLAB Function/1(input)

== system ctrl_TAPM/Thruster control /Thruster 1 ==
  Desired thrust 1 : Inport
  shaft speed : Inport  Port=2
  Constant : Constant  Value=hd2.den{1,1}
  Constant1 : Constant  Value=hd2.num{1,1}
  Delay : Delay  DelayLength=1  InitialCondition=0
  Discrete Transfer Fcn : DiscreteTransferFcn  NumeratorSource=Input port  DenominatorSource=Input port  Denominator=[0.2 1]  SampleTime=0.01  a0EqualsOne=on
      settings: InputPortMap=u0,p1,p3
  Losses (placeholder) : Constant  Value=0
  Propeller Hydrodynamics : Subsystem
  Shaft dynamics : Subsystem
  Thruster control : Subsystem
  "Commanded thrust " : Outport
  Shaft speed : Outport  Port=2
  wires:
  Losses (placeholder)/1 -> Propeller Hydrodynamics/1(env)
  Shaft dynamics/1(n) -> Shaft speed/1, Propeller Hydrodynamics/2(n)
  Propeller Hydrodynamics/2(Qa) -> Delay/1
  Propeller Hydrodynamics/1(Ta) -> "Commanded thrust "/1
  Thruster control/1(Qc) -> Discrete Transfer Fcn/1
  Constant1/1 -> Discrete Transfer Fcn/2
  Constant/1 -> Discrete Transfer Fcn/3
  Discrete Transfer Fcn/1 -> Shaft dynamics/1(Qm)
  shaft speed/1 -> Thruster control/2(n)
  Delay/1 -> Shaft dynamics/2(Qa)
  Desired thrust 1/1 -> Thruster control/1("T_d ")

== system ctrl_TAPM/Thruster control /Thruster 2 ==
  Desired thrust 1 : Inport
  shaft speed : Inport  Port=2
  Constant : Constant  Value=hd2.den{1,1}
  Constant1 : Constant  Value=hd2.num{1,1}
  Delay : Delay  DelayLength=1  InitialCondition=0
  Discrete Transfer Fcn : DiscreteTransferFcn  NumeratorSource=Input port  DenominatorSource=Input port  Denominator=[0.2 1]  SampleTime=0.01  a0EqualsOne=on
      settings: InputPortMap=u0,p1,p3
  Losses (placeholder) : Constant  Value=0
  Propeller Hydrodynamics : Subsystem
  Shaft dynamics : Subsystem
  Thruster control : Subsystem
  "Commanded thrust " : Outport
  Shaft speed : Outport  Port=2
  wires:
  Losses (placeholder)/1 -> Propeller Hydrodynamics/1(env)
  Shaft dynamics/1(n) -> Propeller Hydrodynamics/2(n), Shaft speed/1
  Propeller Hydrodynamics/2(Qa) -> Delay/1
  Thruster control/1(Qc) -> Discrete Transfer Fcn/1
  Discrete Transfer Fcn/1 -> Shaft dynamics/1(Qm)
  Desired thrust 1/1 -> Thruster control/1("T_d ")
  Propeller Hydrodynamics/1(Ta) -> "Commanded thrust "/1
  Constant1/1 -> Discrete Transfer Fcn/2
  Constant/1 -> Discrete Transfer Fcn/3
  shaft speed/1 -> Thruster control/2(n)
  Delay/1 -> Shaft dynamics/2(Qa)

== system ctrl_TAPM/Thruster control /Thruster 3 ==
  Desired thrust 1 : Inport
  shaft speed : Inport  Port=2
  Constant : Constant  Value=hd2.den{1,1}
  Constant1 : Constant  Value=hd2.num{1,1}
  Delay : Delay  DelayLength=1  InitialCondition=0
  Discrete Transfer Fcn : DiscreteTransferFcn  NumeratorSource=Input port  DenominatorSource=Input port  Denominator=[0.2 1]  SampleTime=0.01  a0EqualsOne=on
      settings: InputPortMap=u0,p1,p3
  Losses (placeholder) : Constant  Value=0
  Propeller Hydrodynamics : Subsystem
  Shaft dynamics : Subsystem
  Thruster control : Subsystem
  "Commanded thrust " : Outport
  Shaft speed : Outport  Port=2
  wires:
  Losses (placeholder)/1 -> Propeller Hydrodynamics/1(env)
  Shaft dynamics/1(n) -> Propeller Hydrodynamics/2(n), Shaft speed/1
  Propeller Hydrodynamics/2(Qa) -> Delay/1
  Thruster control/1(Qc) -> Discrete Transfer Fcn/1
  Discrete Transfer Fcn/1 -> Shaft dynamics/1(Qm)
  Desired thrust 1/1 -> Thruster control/1("T_d ")
  Propeller Hydrodynamics/1(Ta) -> "Commanded thrust "/1
  Constant1/1 -> Discrete Transfer Fcn/2
  Constant/1 -> Discrete Transfer Fcn/3
  shaft speed/1 -> Thruster control/2(n)
  Delay/1 -> Shaft dynamics/2(Qa)

== system ctrl_TAPM/Thruster control /Thruster 4 ==
  Desired thrust 1 : Inport
  shaft speed : Inport  Port=2
  Constant : Constant  Value=hd2.den{1,1}
  Constant1 : Constant  Value=hd2.num{1,1}
  Delay : Delay  DelayLength=1  InitialCondition=0
  Discrete Transfer Fcn : DiscreteTransferFcn  NumeratorSource=Input port  DenominatorSource=Input port  Denominator=[0.2 1]  SampleTime=0.01  a0EqualsOne=on
      settings: InputPortMap=u0,p1,p3
  Losses (placeholder) : Constant  Value=0
  Propeller Hydrodynamics : Subsystem
  Shaft dynamics : Subsystem
  Thruster control : Subsystem
  "Commanded thrust " : Outport
  Shaft speed : Outport  Port=2
  wires:
  Losses (placeholder)/1 -> Propeller Hydrodynamics/1(env)
  Shaft dynamics/1(n) -> Propeller Hydrodynamics/2(n), Shaft speed/1
  Propeller Hydrodynamics/2(Qa) -> Delay/1
  Thruster control/1(Qc) -> Discrete Transfer Fcn/1
  Discrete Transfer Fcn/1 -> Shaft dynamics/1(Qm)
  Desired thrust 1/1 -> Thruster control/1("T_d ")
  Propeller Hydrodynamics/1(Ta) -> "Commanded thrust "/1
  Constant1/1 -> Discrete Transfer Fcn/2
  Constant/1 -> Discrete Transfer Fcn/3
  shaft speed/1 -> Thruster control/2(n)
  Delay/1 -> Shaft dynamics/2(Qa)

== system ctrl_TAPM/Thruster control /Thruster 5 ==
  Desired thrust 1 : Inport
  shaft speed : Inport  Port=2
  Constant : Constant  Value=hd2.den{1,1}
  Constant1 : Constant  Value=hd2.num{1,1}
  Delay : Delay  DelayLength=1  InitialCondition=0
  Discrete Transfer Fcn : DiscreteTransferFcn  NumeratorSource=Input port  DenominatorSource=Input port  Denominator=[0.2 1]  SampleTime=0.01  a0EqualsOne=on
      settings: InputPortMap=u0,p1,p3
  Losses (placeholder) : Constant  Value=0
  Propeller Hydrodynamics : Subsystem
  Shaft dynamics : Subsystem
  Thruster control : Subsystem
  "Commanded thrust " : Outport
  Shaft speed : Outport  Port=2
  wires:
  Losses (placeholder)/1 -> Propeller Hydrodynamics/1(env)
  Shaft dynamics/1(n) -> Propeller Hydrodynamics/2(n), Shaft speed/1
  Propeller Hydrodynamics/2(Qa) -> Delay/1
  Thruster control/1(Qc) -> Discrete Transfer Fcn/1
  Discrete Transfer Fcn/1 -> Shaft dynamics/1(Qm)
  Desired thrust 1/1 -> Thruster control/1("T_d ")
  Propeller Hydrodynamics/1(Ta) -> "Commanded thrust "/1
  Constant1/1 -> Discrete Transfer Fcn/2
  Constant/1 -> Discrete Transfer Fcn/3
  shaft speed/1 -> Thruster control/2(n)
  Delay/1 -> Shaft dynamics/2(Qa)

== system ctrl_TAPM/Thruster control /Thruster 6 ==
  Desired thrust 1 : Inport
  shaft speed : Inport  Port=2
  Constant : Constant  Value=hd2.den{1,1}
  Constant1 : Constant  Value=hd2.num{1,1}
  Delay : Delay  DelayLength=1  InitialCondition=0
  Discrete Transfer Fcn : DiscreteTransferFcn  NumeratorSource=Input port  DenominatorSource=Input port  Denominator=[0.2 1]  SampleTime=0.01  a0EqualsOne=on
      settings: InputPortMap=u0,p1,p3
  Losses (placeholder) : Constant  Value=0
  Propeller Hydrodynamics : Subsystem
  Shaft dynamics : Subsystem
  Thruster control : Subsystem
  "Commanded thrust " : Outport
  Shaft speed : Outport  Port=2
  wires:
  Losses (placeholder)/1 -> Propeller Hydrodynamics/1(env)
  Shaft dynamics/1(n) -> Propeller Hydrodynamics/2(n), Shaft speed/1
  Propeller Hydrodynamics/2(Qa) -> Delay/1
  Thruster control/1(Qc) -> Discrete Transfer Fcn/1
  Discrete Transfer Fcn/1 -> Shaft dynamics/1(Qm)
  Desired thrust 1/1 -> Thruster control/1("T_d ")
  Propeller Hydrodynamics/1(Ta) -> "Commanded thrust "/1
  Constant1/1 -> Discrete Transfer Fcn/2
  Constant/1 -> Discrete Transfer Fcn/3
  shaft speed/1 -> Thruster control/2(n)
  Delay/1 -> Shaft dynamics/2(Qa)

== system ctrl_TAPM/TAPM Controller w_observer/PID/DP controller ==
  eta_ref : Inport
  eta : Inport  Port=2
  nu : Inport  Port=3
  Demux : Demux  Outputs=3
  Integrator : Integrator
  Matrix Multiply : Product  Multiplication=Matrix(*)
  Matrix Multiply1 : Product  Multiplication=Matrix(*)
  Matrix Multiply2 : Product  Multiplication=Matrix(*)
  Mux : Mux  Inputs=3
  Sum1 : Sum  Inputs=|+-  SaturateOnIntegerOverflow=on  InputSameDT=on  OutDataTypeStr=Inherit: Same as first input
  Sum2 : Sum  Inputs=+-|  SaturateOnIntegerOverflow=on  InputSameDT=on  OutDataTypeStr=Inherit: Same as first input
  Sum3 : Sum  Inputs=|++  SaturateOnIntegerOverflow=on  InputSameDT=on  OutDataTypeStr=Inherit: Same as first input
  Transposed rotation matrix in yaw1 : marine_gnc/Models/ Kinematics/Transposed rotation  matrix in yaw
  "[-inf inf] to [-pi pi]" : marine_gnc/Utilities/Math Operations/[-inf inf] to [-pi pi]
  "[-inf inf] to [-pi pi]1" : marine_gnc/Utilities/Math Operations/[-inf inf] to [-pi pi]
  yaw angle : Fcn  Expr=u(3)
  tau : Outport  InitialOutput=0
  wires:
  "[-inf inf] to [-pi pi]1"/1 -> Transposed rotation matrix in yaw1/1
  yaw angle/1 -> "[-inf inf] to [-pi pi]1"/1  "psi"
  Mux/1 -> Transposed rotation matrix in yaw1/2
  Demux/1 -> Mux/1
  Demux/2 -> Mux/2
  "[-inf inf] to [-pi pi]"/1 -> Mux/3
  Sum2/1 -> Demux/1  "regulation error"
  Demux/3 -> "[-inf inf] to [-pi pi]"/1
  eta_ref/1 -> Sum2/1
  Sum1/1 -> tau/1
  eta/1 -> Sum2/2, yaw angle/1
  nu/1 -> Matrix Multiply2/2
  Matrix Multiply2/1 -> Sum1/2
  Matrix Multiply/1 -> Sum3/1
  Sum3/1 -> Sum1/1
  Matrix Multiply1/1 -> Sum3/2
  Transposed rotation matrix in yaw1/1 -> Matrix Multiply/2, Integrator/1
  [K_p] -> Matrix Multiply/1
  Integrator/1 -> Matrix Multiply1/2
  [K_i] -> Matrix Multiply1/1
  [K_d] -> Matrix Multiply2/1

== system ctrl_TAPM/TAPM Controller w_observer/PID/DP controller1 ==
  eta_ref : Inport
  eta : Inport  Port=2
  nu : Inport  Port=3
  Demux : Demux  Outputs=3
  Integrator : Integrator
  Matrix Multiply : Product  Multiplication=Matrix(*)
  Matrix Multiply1 : Product  Multiplication=Matrix(*)
  Matrix Multiply2 : Product  Multiplication=Matrix(*)
  Mux : Mux  Inputs=3
  Sum1 : Sum  Inputs=|+-  SaturateOnIntegerOverflow=on  InputSameDT=on  OutDataTypeStr=Inherit: Same as first input
  Sum2 : Sum  Inputs=+-|  SaturateOnIntegerOverflow=on  InputSameDT=on  OutDataTypeStr=Inherit: Same as first input
  Sum3 : Sum  Inputs=|++  SaturateOnIntegerOverflow=on  InputSameDT=on  OutDataTypeStr=Inherit: Same as first input
  Transposed rotation matrix in yaw1 : marine_gnc/Models/ Kinematics/Transposed rotation  matrix in yaw
  "[-inf inf] to [-pi pi]" : marine_gnc/Utilities/Math Operations/[-inf inf] to [-pi pi]
  "[-inf inf] to [-pi pi]1" : marine_gnc/Utilities/Math Operations/[-inf inf] to [-pi pi]
  yaw angle : Fcn  Expr=u(3)
  tau : Outport  InitialOutput=0
  wires:
  "[-inf inf] to [-pi pi]1"/1 -> Transposed rotation matrix in yaw1/1
  yaw angle/1 -> "[-inf inf] to [-pi pi]1"/1  "psi"
  Mux/1 -> Transposed rotation matrix in yaw1/2
  Demux/1 -> Mux/1
  Demux/2 -> Mux/2
  "[-inf inf] to [-pi pi]"/1 -> Mux/3
  Sum2/1 -> Demux/1  "regulation error"
  Demux/3 -> "[-inf inf] to [-pi pi]"/1
  eta_ref/1 -> Sum2/1
  Sum1/1 -> tau/1
  eta/1 -> Sum2/2, yaw angle/1
  nu/1 -> Matrix Multiply2/2
  Matrix Multiply2/1 -> Sum1/2
  Matrix Multiply/1 -> Sum3/1
  Sum3/1 -> Sum1/1
  Matrix Multiply1/1 -> Sum3/2
  Transposed rotation matrix in yaw1/1 -> Matrix Multiply/2, Integrator/1
  [K_p_outside] -> Matrix Multiply/1
  Integrator/1 -> Matrix Multiply1/2
  [K_i_outside] -> Matrix Multiply1/1
  [K_d_outside] -> Matrix Multiply2/1
